simulink model "q2"  (R2019a)
settings: Solver=VariableStepAuto  StartTime=0.0  StopTime=10.0  RelTol=1e-3
settings Model: Creator=peedr  LastModifiedBy=peedr

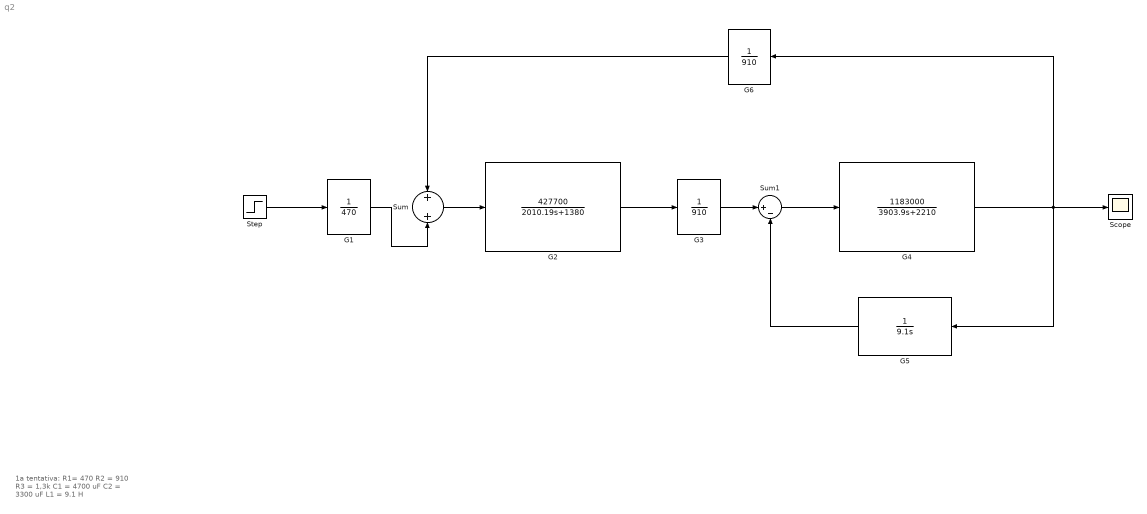
== system q2 ==
  note: 1a tentativa:
      | R1= 470
      | R2 = 910
      | R3 = 1,3k
      | C1 = 4700 uF
      | C2 = 3300 uF
      | L1 = 9.1 H
  G1 : TransferFcn  Denominator=[470]
  G2 : TransferFcn  Numerator=[427700]  Denominator=[2010.19 1380]
  G3 : TransferFcn  Denominator=[910]
  G4 : TransferFcn  Numerator=[1183000]  Denominator=[3903.9 2210]
  G5 : TransferFcn  Denominator=[9.1 0]
  G6 : TransferFcn  Denominator=[910]
  Scope : Scope
  Step : Step  SampleTime=0
  Sum : Sum
  Sum1 : Sum  Inputs=|+-
  wires:
  G2/1 -> G3/1
  Sum/1 -> G2/1
  G3/1 -> Sum1/1
  Sum1/1 -> G4/1
  G4/1 -> Scope/1, G6/1, G5/1
  G6/1 -> Sum/1
  G1/1 -> Sum/2
  G5/1 -> Sum1/2
  Step/1 -> G1/1
